simulink model "model"  (R2020b)
settings: Solver=VariableStepAuto  StartTime=0.0  StopTime=10.0  RelTol=1e-3
settings Model: Creator=Vrunda M Balgi  LastModifiedBy=Vrunda M Balgi

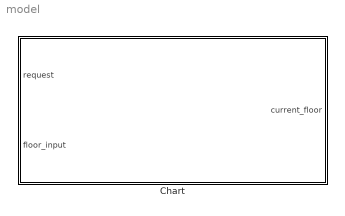
== system model ==
  Chart : Stateflow chart  TreatAsAtomicUnit=on

== stateflow chart model/Chart ==
  state Idle
  state PrepareLift
    entry:
    door_close = 1;
  state LiftAction
    (history)
    state Floor1
      entry:
      current_floor = 1;
      (default) -> (junction 89)
      (junction 89) -> (junction 90) [order 1] : [current_floor == floor_input]
      (junction 89) -> (junction 91) [order 2]
      (junction 90) -> (junction 92) : {door_close = 0;}
      (junction 92) -> (junction 91)
      (junction 91) -> (junction 93)
    state Floor2
      entry:
      current_floor = 2;
      (default) -> (junction 94)
      (junction 94) -> (junction 97) [order 1] : [current_floor == floor_input]
      (junction 94) -> (junction 95) [order 2]
      (junction 97) -> (junction 103) : {door_close = 0;}
      (junction 103) -> (junction 95)
      (junction 95) -> (junction 102)
    state Floor3
      entry:
      current_floor = 3;
      (default) -> (junction 117)
      (junction 117) -> (junction 120) [order 1] : [current_floor == floor_input]
      (junction 117) -> (junction 118) [order 2]
      (junction 120) -> (junction 126) : {door_close = 0;}
      (junction 126) -> (junction 118)
      (junction 118) -> (junction 125)
    state Floor4
      entry:
      current_floor = 4;
      (default) -> (junction 128)
      (junction 128) -> (junction 131) [order 1] : [current_floor == floor_input]
      (junction 128) -> (junction 129) [order 2]
      (junction 131) -> (junction 137) : {door_close = 0;}
      (junction 137) -> (junction 129)
      (junction 129) -> (junction 136)
    state Floor5
      entry:
      current_floor = 5;
      (default) -> (junction 139)
      (junction 139) -> (junction 142) [order 1] : [current_floor == floor_input]
      (junction 139) -> (junction 140) [order 2]
      (junction 142) -> (junction 148) : {door_close = 0;}
      (junction 148) -> (junction 140)
      (junction 140) -> (junction 147)
    (default) -> Floor1
    Floor1 -> Floor2 : [floor_input>current_floor]
    Floor2 -> Floor1 [order 2] : [floor_input<current_floor]
    Floor2 -> Floor3 [order 1] : [floor_input>current_floor]
    Floor3 -> Floor2 [order 2] : [floor_input<current_floor]
    Floor3 -> Floor4 [order 1] : [floor_input>current_floor]
    Floor4 -> Floor3 [order 2] : [floor_input<current_floor]
    Floor4 -> Floor5 [order 1] : [floor_input>current_floor]
    Floor5 -> Floor4 : [floor_input<current_floor]
  (default) -> Idle
  Idle -> PrepareLift : [request==1 && floor_input~=0]
  PrepareLift -> LiftAction
  data: door_close local; request input; floor_input input; current_floor output
